simulink model "EstHeatingSys"  (R2017a)
settings: Solver=FixedStepAuto  StartTime=0.0  StopTime=100  FixedStep=0.1  MaxStep=0.1  RelTol=1e-3
libraries: simulink x1
settings Model: Creator=xiaodong  LastModifiedBy=xiaodong

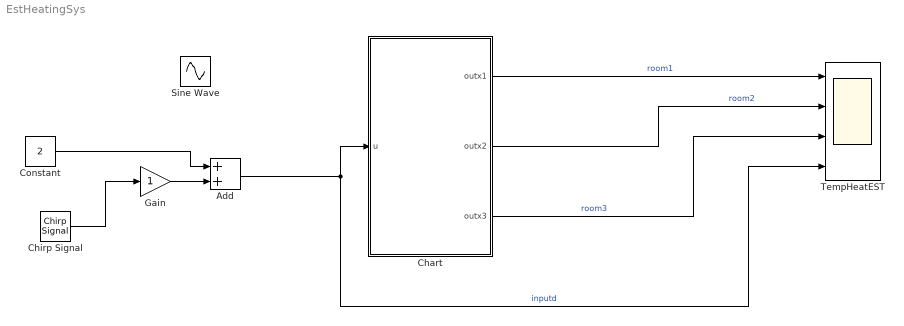
== system EstHeatingSys ==
  Add : Sum
  Chart : Stateflow chart  TreatAsAtomicUnit=on
  Chirp Signal : simulink/Sources/Chirp Signal  f1=0.001  T=1000  f2=0.1
  Constant : Constant  Value=2
  Gain : Gain
  Sine Wave : Sin  Amplitude=2  Bias=6  Frequency=0.05  SampleTime=0
  TempHeatEST : Scope  NumInputPorts=4
  wires:
  Add/1 -> TempHeatEST/4, Chart/1(u)  "inputd"
  Gain/1 -> Add/2
  Chirp Signal/1 -> Gain/1
  Constant/1 -> Add/1
  Chart/3(outx3) -> TempHeatEST/3  "room3"
  Chart/2(outx2) -> TempHeatEST/2  "room2"
  Chart/1(outx1) -> TempHeatEST/1  "room1"

== stateflow chart EstHeatingSys/Chart ==
  state sys
    state X1 [parallel]
      settings: executionOrder=1
      state E
        entry:
        %x1 = A10(1) *x1 +  A10(2)* x2 +...
        %    A10(3)*x3 +  A10(4)*u + A10(5);
        H(1)=0;
      state on1
        entry:
        %x1 =A11(1) *x1 +  A11(2)* x2 +...
        %   A11(3)*x3  +  A11(4)*u + A11(5);
        H(1)=1;
      state off1
        entry:
        %x1 = A10(1) *x1 +  A10(2)* x2 +...
        %   A10(3)*x3 +  A10(4)*u + A10(5);
        H(1)=0;
      (default) -> E
      E -> sys.X1.on1 : [-0.0636*x1-0.0005*x2+0.0013*x3+1>=0 ...
          |  && 0.4761*x1+0.0005*x2-0.4764*x3+1<=0]
      sys.X1.off1 -> E [order 2] : [-0.3300*x1+0.3297*x2+0.0013*x3+1<=0&&...
          | -0.0004*x1-0.0638*x2+0.0019*x3 + 1>=0]
      sys.X1.on1 -> E [order 2] : [-0.3300*x1+0.3297*x2+0.0013*x3+1<=0&&...
          | -0.0004*x1-0.0638*x2+0.0019*x3 + 1>=0]
      sys.X1.off1 -> sys.X1.on1 [order 1] : [-0.0511*x1-0.0002*x2 + 0.0014*x3 + 1>=0]
      sys.X1.on1 -> sys.X1.off1 [order 1] : [-0.0479*x1-0.0004*x2+0.0010*x3+1<=0]
    state X2 [parallel]
      settings: executionOrder=2
      state E2
        entry:
        %x2 = A20(1) *x1 +  A20(2)* x2 +...
        %    A20(3)*x3 +  A20(4)*u + A20(5);
        H(2)=0;
      state on2
        entry:
        %x2 =A21(1) *x1 +  A21(2)* x2 +...
        %    A21(3)*x3  +  A21(4)*u + A21(5);
        H(2)=1;
      state off2
        entry:
        %x2 = A20(1) *x1 +  A20(2)* x2 +...
        %    A20(3)*x3 +  A20(4)*u + A20(5);
        H(2)=0;
      E2 -> on2 : [-0.3300*x1+0.3297*x2+0.0013*x3+1<=0&&...
          | -0.0004*x1-0.0638*x2+0.0019*x3 + 1>=0]
      off2 -> E2 [order 2] : [-0.0009*x1-0*x2-0.0660*x3+1>=0&&...
          |  0.0032*x1-0.4794*x2+0.4760*x3+1<=0]
      on2 -> E2 [order 2] : [-0.0009*x1-0*x2-0.0660*x3+1>=0&&...
          |  0.0032*x1-0.4794*x2+0.4760*x3+1<=0]
      (default) -> on2
      off2 -> on2 [order 1] : [-0.0012*x1-0.0533*x2+0.0019*x3+1>=0]
      on2 -> off2 [order 1] : [-0.0008*x1-0.0481*x2+0.0016*x3+1<=0]
    state X3 [parallel]
      settings: executionOrder=3
      state E3
        entry:
        %x3 = A30(1) *x1 +  A30(2)* x2 +...
        %    A30(3)*x3 +  A30(4)*u + A30(5);
        H(3)=0;
      state on1
        entry:
        %x3 =A31(1) *x1 +  A31(2)* x2 +...
        %    A31(3)*x3  +  A31(4)*u + A31(5);
        H(3)=1;
      state off1
        entry:
        %x3 = A30(1) *x1 +  A30(2)* x2 +...
        %   A30(3)*x3 +  A30(4)*u + A30(5);
        H(3)=0;
      E3 -> sys.X3.on1 : [-0.0009*x1-0*x2-0.0660*x3+1>=0&&...
          |  0.0032*x1-0.4794*x2+0.4760*x3+1<=0]
      (default) -> E3
      sys.X3.off1 -> E3 [order 2] : [ 0.4831*x1-0.0006*x2-0.4814*x3+1<=0&&...
          | -0.0637*x1-0.0005*x2+0.0013*x3+1>=0]
      sys.X3.on1 -> E3 [order 2] : [-0.0636*x1-0.0005*x2+0.0013*x3+1>=0 ...
          |  && 0.4761*x1+0.0005*x2-0.4764*x3+1<=0]
      sys.X3.off1 -> sys.X3.on1 [order 1] : [ 0.0015*x1+0.0035*x2-0.0574*x3+1>=0]
      sys.X3.on1 -> sys.X3.off1 [order 1] : [ 0.0010*x1-0.0014*x2-0.0450*x3+1<=0]
    state XX [parallel]
      entry:
      outx1 = xn1;
      outx2 = xn2;
      outx3 = xn3;
      if H(1) == 1
      xn1 =A11(1) *x1 +  A11(2)* x2 + A11(3)*x3  +  A11(4)*u + A11(5);
      end
      if H(1) == 0
      xn1 = A10(1) *x1 +  A10(2)* x2 +A10(3)*x3 +  A10(4)*u + A10(5);
      end
      if H(2) ==1
      xn2 =A21(1) *x1 +  A21(2)* x2 + A21(3)*x3  +  A21(4)*u + A21(5);
      end
      if H(2) == 0
      xn2 = A20(1) *x1 +  A20(2)* x2 + A20(3)*x3 +  A20(4)*u + A20(5);
      end
      if H(3)==1
      xn3 =A31(1) *x1 +  A31(2)* x2 +A31(3)*x3  +  A31(4)*u + A31(5);
      end
      if H(3) == 0
      xn3 = A30(1) *x1 +  A30(2)* x2 +A30(3)*x3 +  A30(4)*u + A30(5);
      end
      %xn1 = A(1,1)*x1+A(1,2)*x2 + A(1,3)*x3+H(1)*B(1,1)+H(2)*B(1,2)+H(3)*B(1,3)+B(1,4)*u;
      %xn2 = A(2,1)*x1+A(2,2)*x2 + A(2,3)*x3+H(1)*B(2,1)+H(2)*B(2,2)+H(3)*B(2,3)+B(2,4)*u;
      %xn3 = A(3,1)*x1+A(3,2)*x2 + A(3,3)*x3+H(1)*B(3,1)+H(2)*B(3,2)+H(3)*B(3,3)+B(3,4)*u;
      x1 = xn1;
      x2 = xn2;
      x3 = xn3;
      during:
      outx1 = xn1;
      outx2 = xn2;
      outx3 = xn3;
      if H(1) ==1
      xn1 =A11(1) *x1 +  A11(2)* x2 + A11(3)*x3  +  A11(4)*u + A11(5);
      end
      if H(1) ==0
      xn1 = A10(1) *x1 +  A10(2)* x2 +A10(3)*x3 +  A10(4)*u + A10(5);
      end
      if H(2) ==1
      xn2 =A21(1) *x1 +  A21(2)* x2 + A21(3)*x3  +  A21(4)*u + A21(5);
      end
      if H(2)==0
      xn2 = A20(1) *x1 +  A20(2)* x2 + A20(3)*x3 +  A20(4)*u + A20(5);
      end
      if H(3)==1
      xn3 =A31(1) *x1 +  A31(2)* x2 +A31(3)*x3  +  A31(4)*u + A31(5);
      end
      if H(3)==0
      xn3 = A30(1) *x1 +  A30(2)* x2 +A30(3)*x3 +  A30(4)*u + A30(5);
      end
      %xn1 = A(1,1)*x1+A(1,2)*x2 + A(1,3)*x3+H(1)*B(1,1)+H(2)*B(1,2)+H(3)*B(1,3)+B(1,4)*u;
      %xn2 = A(2,1)*x1+A(2,2)*x2 + A(2,3)*x3+H(1)*B(2,1)+H(2)*B(2,2)+H(3)*B(2,3)+B(2,4)*u;
      %xn3 = A(3,1)*x1+A(3,2)*x2 + A(3,3)*x3+H(1)*B(3,1)+H(2)*B(3,2)+H(3)*B(3,3)+B(3,4)*u;
      x1 = xn1;
      x2 = xn2;
      x3 = xn3;
      settings: executionOrder=4
  (default) -> sys : {x1=14; x2=14; x3= 14; outx1 = x1; outx2 = x2; outx3 =x3; xn1 = x1; xn2 = x2; xn3 = x3;}
  data: A10 constant double size=5 =A1(:,1); u input; A11 constant double size=5 =A1(:,2); A20 constant double size=5 =A2(:,1); A21 constant double size=5 =A2(:,2); A30 constant double size=5 =A3(:,1); A31 constant double size=5 =A3(:,2); H local size=3 =[0,0,0]'; B constant double size=3,4 =ones(3,4); xn1 local =14; xn2 local =14; xn3 local =14; x1 local; x2 local; x3 local; outx1 output =16; outx2 output =12; outx3 output =15; A constant double size=3,3 =ones(3,3)
  data x1 settings: updateMethod=SF_CONTINUOUS_TIME_DATA
  data x2 settings: updateMethod=SF_CONTINUOUS_TIME_DATA
  data x3 settings: updateMethod=SF_CONTINUOUS_TIME_DATA
